simulink model "VMC_Integration"  (R2024a)
settings: Solver=FixedStepDiscrete  StartTime=0.0  StopTime=10.0  FixedStep=0.005  RelTol=1e-3
undefined symbols (not defined in the file): Degree_To_Rad_Factor
libraries: simulink x24, slpidlib x5
(part 2 of 3)

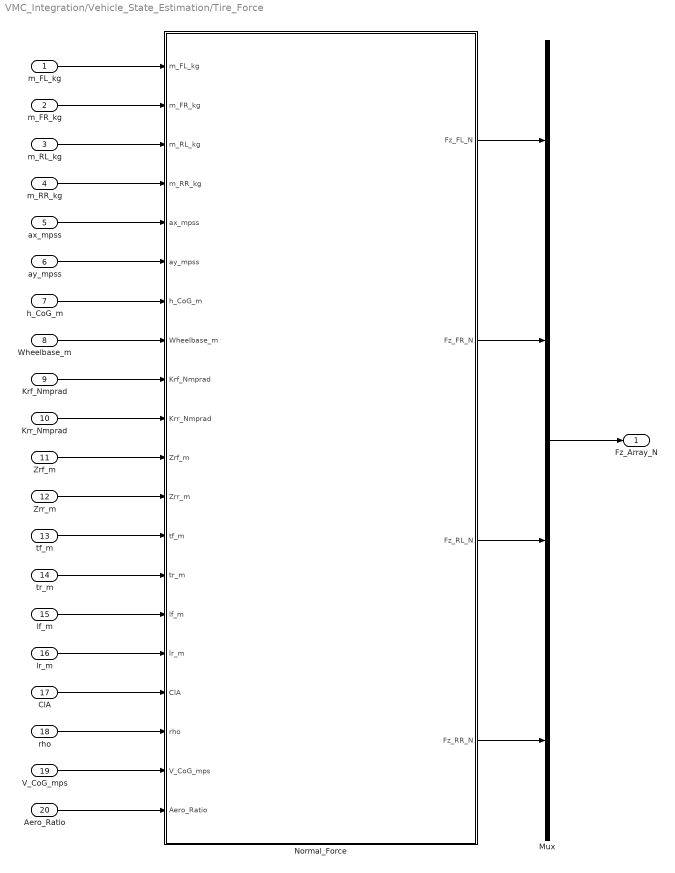
== system VMC_Integration/Vehicle_State_Estimation/Tire_Force ==
  m_FL_kg : Inport
  m_FR_kg : Inport  Port=2
  m_RL_kg : Inport  Port=3
  m_RR_kg : Inport  Port=4
  ax_mpss : Inport  Port=5
  ay_mpss : Inport  Port=6
  h_CoG_m : Inport  Port=7
  Wheelbase_m : Inport  Port=8
  Krf_Nmprad : Inport  Port=9
  Krr_Nmprad : Inport  Port=10
  Zrf_m : Inport  Port=11
  Zrr_m : Inport  Port=12
  tf_m : Inport  Port=13
  tr_m : Inport  Port=14
  lf_m : Inport  Port=15
  lr_m : Inport  Port=16
  ClA : Inport  Port=17
  rho : Inport  Port=18
  V_CoG_mps : Inport  Port=19
  Aero_Ratio : Inport  Port=20
  Mux : Mux
  Normal_Force : Subsystem
  Fz_Array_N : Outport
  wires:
  Normal_Force/1(Fz_FL_N) -> Mux/1
  Normal_Force/2(Fz_FR_N) -> Mux/2
  Normal_Force/3(Fz_RL_N) -> Mux/3
  Normal_Force/4(Fz_RR_N) -> Mux/4
  Mux/1 -> Fz_Array_N/1
  m_FL_kg/1 -> Normal_Force/1(m_FL_kg)
  m_FR_kg/1 -> Normal_Force/2(m_FR_kg)
  m_RL_kg/1 -> Normal_Force/3(m_RL_kg)
  m_RR_kg/1 -> Normal_Force/4(m_RR_kg)
  ax_mpss/1 -> Normal_Force/5(ax_mpss)
  ay_mpss/1 -> Normal_Force/6(ay_mpss)
  h_CoG_m/1 -> Normal_Force/7(h_CoG_m)
  Wheelbase_m/1 -> Normal_Force/8(Wheelbase_m)
  Krf_Nmprad/1 -> Normal_Force/9(Krf_Nmprad)
  Krr_Nmprad/1 -> Normal_Force/10(Krr_Nmprad)
  Zrf_m/1 -> Normal_Force/11(Zrf_m)
  Zrr_m/1 -> Normal_Force/12(Zrr_m)
  tf_m/1 -> Normal_Force/13(tf_m)
  tr_m/1 -> Normal_Force/14(tr_m)
  lf_m/1 -> Normal_Force/15(lf_m)
  lr_m/1 -> Normal_Force/16(lr_m)
  ClA/1 -> Normal_Force/17(ClA)
  rho/1 -> Normal_Force/18(rho)
  V_CoG_mps/1 -> Normal_Force/19(V_CoG_mps)
  Aero_Ratio/1 -> Normal_Force/20(Aero_Ratio)

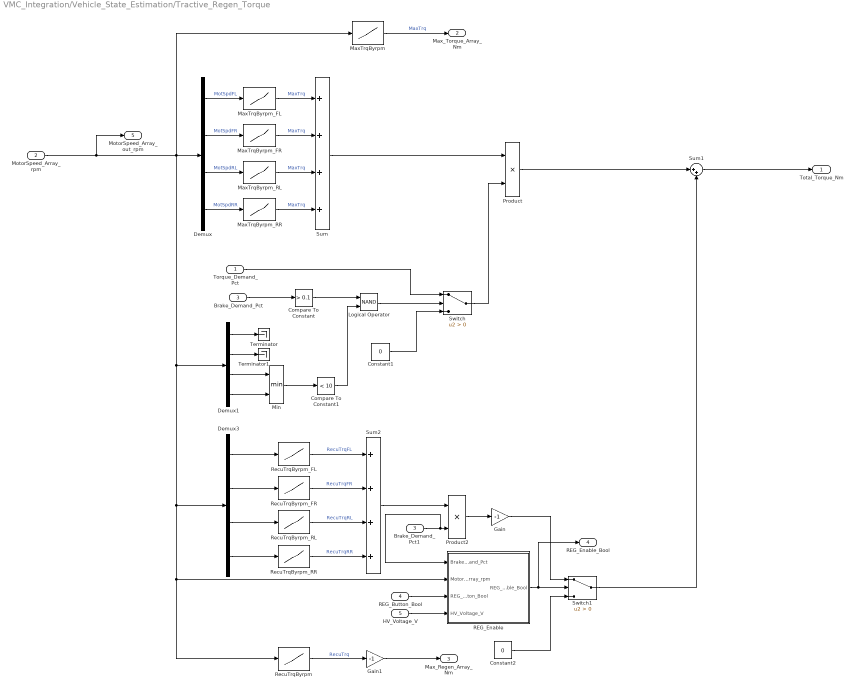
== system VMC_Integration/Vehicle_State_Estimation/Tractive_Regen_Torque ==
  Torque_Demand_Pct : Inport  OutDataTypeStr=single
  MotorSpeed_Array_rpm : Inport  Port=2  OutDataTypeStr=single
  Brake_Demand_Pct : Inport  Port=3  OutDataTypeStr=single
  REG_Button_Bool : Inport  Port=4
  HV_Voltage_V : Inport  Port=5
  Brake_Demand_Pct1 : InportShadow  Port=3  OutDataTypeStr=single
  Compare To Constant : simulink/Logic and Bit Operations/Compare To Constant  relop=>  const=0.1  OutDataTypeStr=boolean
  Compare To Constant1 : simulink/Logic and Bit Operations/Compare To Constant  relop=<  const=10  OutDataTypeStr=boolean
  Constant1 : Constant  Value=0  OutDataTypeStr=single  SampleTime=-1
  Constant2 : Constant  Value=0  OutDataTypeStr=single  SampleTime=-1
  Demux : Demux
  Demux1 : Demux
  Demux3 : Demux
  Gain : Gain  Gain=-1  ParamDataTypeStr=single  OutDataTypeStr=single
  Gain1 : Gain  Gain=-1  ParamDataTypeStr=single  OutDataTypeStr=single
  Logical Operator : Logic  Operator=NAND  AllPortsSameDT=off  OutDataTypeStr=boolean
  MaxTrqByrpm : Lookup_n-D  NumberOfTableDimensions=1  BreakpointsForDimension1=[0,16000,19999,20000]  BreakpointsForDimension1DataTypeStr=single  Table=[21,21,13,0]  TableDataTypeStr=single  IntermediateResultsDataTypeStr=single  InternalRulePriority=Speed  OutDataTypeStr=single  RndMeth=Simplest  FractionDataTypeStr=single
  MaxTrqByrpm_FL : Lookup_n-D  NumberOfTableDimensions=1  BreakpointsForDimension1=[0,16000,19999,20000]  BreakpointsForDimension1DataTypeStr=single  Table=[21,21,13,0]  TableDataTypeStr=single  IntermediateResultsDataTypeStr=single  InternalRulePriority=Speed  OutDataTypeStr=single  RndMeth=Simplest  FractionDataTypeStr=single
  MaxTrqByrpm_FR : Lookup_n-D  NumberOfTableDimensions=1  BreakpointsForDimension1=[0,16000,19999,20000]  BreakpointsForDimension1DataTypeStr=single  Table=[21,21,13,0]  TableDataTypeStr=single  IntermediateResultsDataTypeStr=single  InternalRulePriority=Speed  OutDataTypeStr=single  RndMeth=Simplest  FractionDataTypeStr=single
  MaxTrqByrpm_RL : Lookup_n-D  NumberOfTableDimensions=1  BreakpointsForDimension1=[0,16000,19999,20000]  BreakpointsForDimension1DataTypeStr=single  Table=[21,21,13,0]  TableDataTypeStr=single  IntermediateResultsDataTypeStr=single  InternalRulePriority=Speed  OutDataTypeStr=single  RndMeth=Simplest  FractionDataTypeStr=single
  MaxTrqByrpm_RR : Lookup_n-D  NumberOfTableDimensions=1  BreakpointsForDimension1=[0,16000,19999,20000]  BreakpointsForDimension1DataTypeStr=single  Table=[21,21,13,0]  TableDataTypeStr=single  IntermediateResultsDataTypeStr=single  InternalRulePriority=Speed  OutDataTypeStr=single  RndMeth=Simplest  FractionDataTypeStr=single
  Min : MinMax  Inputs=2
  Product : Product
  Product2 : Product  OutDataTypeStr=single
  REG_Enable : Subsystem
  RecuTrqByrpm : Lookup_n-D  NumberOfTableDimensions=1  BreakpointsForDimension1=[0,1500,5000,20000]  BreakpointsForDimension1DataTypeStr=single  Table=[0,0,17,17]  TableDataTypeStr=single  IntermediateResultsDataTypeStr=single  InternalRulePriority=Speed  OutDataTypeStr=single  RndMeth=Simplest  FractionDataTypeStr=single
  RecuTrqByrpm_FL : Lookup_n-D  NumberOfTableDimensions=1  BreakpointsForDimension1=[0,1500,5000,20000]  BreakpointsForDimension1DataTypeStr=single  Table=[0,0,17,17]  TableDataTypeStr=single  IntermediateResultsDataTypeStr=single  InternalRulePriority=Speed  OutDataTypeStr=single  RndMeth=Simplest  FractionDataTypeStr=single
  RecuTrqByrpm_FR : Lookup_n-D  NumberOfTableDimensions=1  BreakpointsForDimension1=[0,1500,5000,20000]  BreakpointsForDimension1DataTypeStr=single  Table=[0,0,17,17]  TableDataTypeStr=single  IntermediateResultsDataTypeStr=single  InternalRulePriority=Speed  OutDataTypeStr=single  RndMeth=Simplest  FractionDataTypeStr=single
  RecuTrqByrpm_RL : Lookup_n-D  NumberOfTableDimensions=1  BreakpointsForDimension1=[0,1500,5000,20000]  BreakpointsForDimension1DataTypeStr=single  Table=[0,0,17,17]  TableDataTypeStr=single  IntermediateResultsDataTypeStr=single  InternalRulePriority=Speed  OutDataTypeStr=single  RndMeth=Simplest  FractionDataTypeStr=single
  RecuTrqByrpm_RR : Lookup_n-D  NumberOfTableDimensions=1  BreakpointsForDimension1=[0,1500,5000,20000]  BreakpointsForDimension1DataTypeStr=single  Table=[0,0,17,17]  TableDataTypeStr=single  IntermediateResultsDataTypeStr=single  InternalRulePriority=Speed  OutDataTypeStr=single  RndMeth=Simplest  FractionDataTypeStr=single
  Sum : Sum  Inputs=++++
  Sum1 : Sum  Inputs=|++  OutDataTypeStr=single  AccumDataTypeStr=single
  Sum2 : Sum  Inputs=++++  AccumDataTypeStr=single
  Switch : Switch  Criteria=u2 > Threshold  OutDataTypeStr=single  SaturateOnIntegerOverflow=off  InputSameDT=off
  Switch1 : Switch  Criteria=u2 > Threshold  OutDataTypeStr=single  SaturateOnIntegerOverflow=off  InputSameDT=off
  Terminator : Terminator
  Terminator1 : Terminator
  Total_Torque_Nm : Outport
  Max_Torque_Array_Nm : Outport  Port=2
  Max_Regen_Array_Nm : Outport  Port=3
  REG_Enable_Bool : Outport  Port=4
  MotorSpeed_Array_out_rpm : Outport  Port=5
  wires:
  Demux/1 -> MaxTrqByrpm_FL/1  "MotSpdFL"
  Demux/2 -> MaxTrqByrpm_FR/1  "MotSpdFR"
  Demux/3 -> MaxTrqByrpm_RL/1  "MotSpdRL"
  Demux/4 -> MaxTrqByrpm_RR/1  "MotSpdRR"
  MaxTrqByrpm_FL/1 -> Sum/1  "MaxTrq"
  MaxTrqByrpm_FR/1 -> Sum/2  "MaxTrq"
  MaxTrqByrpm_RL/1 -> Sum/3  "MaxTrq"
  MaxTrqByrpm_RR/1 -> Sum/4  "MaxTrq"
  Sum/1 -> Product/1
  MaxTrqByrpm/1 -> Max_Torque_Array_Nm/1  "MaxTrq"
  Demux1/2 -> Terminator1/1
  Demux1/3 -> Min/1
  Switch/1 -> Product/2
  Constant1/1 -> Switch/3
  Logical Operator/1 -> Switch/2
  Demux1/4 -> Min/2
  Compare To Constant/1 -> Logical Operator/1
  Min/1 -> Compare To Constant1/1
  Demux1/1 -> Terminator/1
  Compare To Constant1/1 -> Logical Operator/2
  MotorSpeed_Array_rpm/1 -> MotorSpeed_Array_out_rpm/1, Demux1/1, RecuTrqByrpm/1, REG_Enable/2(MotorSpeed_Array_rpm), Demux3/1, MaxTrqByrpm/1, Demux/1
  Torque_Demand_Pct/1 -> Switch/1
  Brake_Demand_Pct/1 -> Compare To Constant/1
  REG_Enable/1(REG_Enable_Bool) -> REG_Enable_Bool/1, Switch1/2
  Gain/1 -> Switch1/1
  Brake_Demand_Pct1/1 -> REG_Enable/1(Brake_Demand_Pct), Product2/2
  Demux3/2 -> RecuTrqByrpm_FR/1
  Demux3/3 -> RecuTrqByrpm_RL/1
  Demux3/1 -> RecuTrqByrpm_FL/1
  Sum2/1 -> Product2/1
  Product2/1 -> Gain/1
  RecuTrqByrpm_RL/1 -> Sum2/3  "RecuTrqRL"
  RecuTrqByrpm_FL/1 -> Sum2/1  "RecuTrqFL"
  RecuTrqByrpm_FR/1 -> Sum2/2  "RecuTrqFR"
  Demux3/4 -> RecuTrqByrpm_RR/1
  RecuTrqByrpm_RR/1 -> Sum2/4  "RecuTrqRR"
  Constant2/1 -> Switch1/3
  REG_Button_Bool/1 -> REG_Enable/3(REG_Button_Bool)
  HV_Voltage_V/1 -> REG_Enable/4(HV_Voltage_V)
  Product/1 -> Sum1/1
  Sum1/1 -> Total_Torque_Nm/1
  Switch1/1 -> Sum1/2
  RecuTrqByrpm/1 -> Gain1/1  "RecuTrq"
  Gain1/1 -> Max_Regen_Array_Nm/1

== system VMC_Integration/Vehicle_State_Estimation/Velocity_Estimation ==
  IMU_YawRate_radps : Inport
  OS_Vx_kph : Inport  Port=2
  OS_Vy_kph : Inport  Port=3
  OS_X_Distance_m : Inport  Port=4
  OS_Y_Distance_m : Inport  Port=5
  CoG_Linear_Velocity_Calculation : MATLAB Function  TreatAsAtomicUnit=on
  CoG_Vx_mps : Outport
  CoG_Vy_mps : Outport  Port=2
  CoG_V_mps : Outport  Port=3
  OS_V_mps : Outport  Port=4
  wires:
  IMU_YawRate_radps/1 -> CoG_Linear_Velocity_Calculation/1(Actual_Yaw_Rate)
  OS_Vx_kph/1 -> CoG_Linear_Velocity_Calculation/2(OS_Vx)
  OS_Vy_kph/1 -> CoG_Linear_Velocity_Calculation/3(OS_Vy)
  OS_X_Distance_m/1 -> CoG_Linear_Velocity_Calculation/4(OS_X_Distance)
  OS_Y_Distance_m/1 -> CoG_Linear_Velocity_Calculation/5(OS_Y_Distance)
  CoG_Linear_Velocity_Calculation/1(CoG_Vx) -> CoG_Vx_mps/1
  CoG_Linear_Velocity_Calculation/2(CoG_Vy) -> CoG_Vy_mps/1
  CoG_Linear_Velocity_Calculation/3(CoG_V) -> CoG_V_mps/1
  CoG_Linear_Velocity_Calculation/4(OS_V) -> OS_V_mps/1

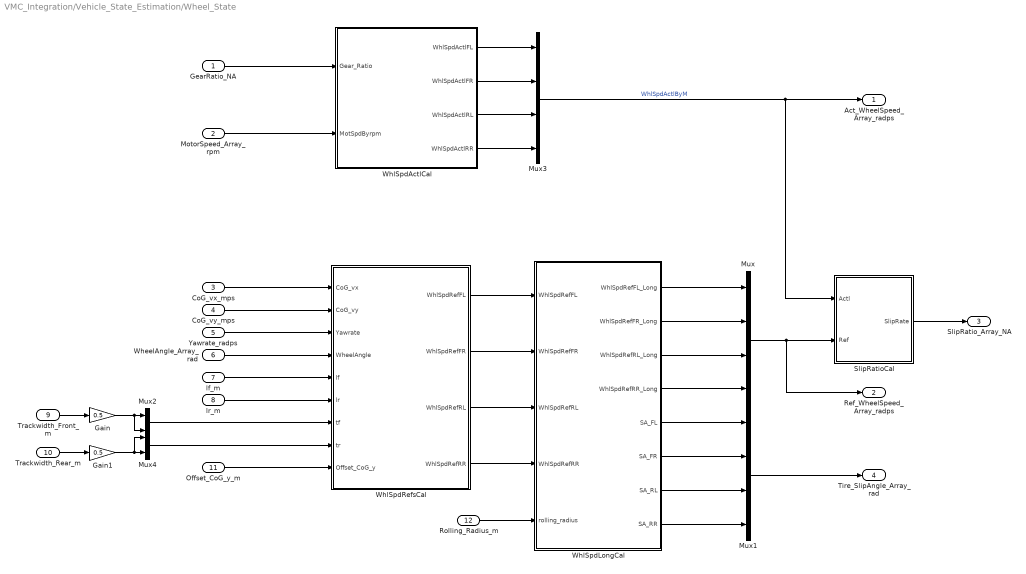
== system VMC_Integration/Vehicle_State_Estimation/Wheel_State ==
  GearRatio_NA : Inport
  MotorSpeed_Array_rpm : Inport  Port=2  PortDimensions=[4,1]
  CoG_vx_mps : Inport  Port=3
  CoG_vy_mps : Inport  Port=4
  Yawrate_radps : Inport  Port=5
  WheelAngle_Array_rad : Inport  Port=6  PortDimensions=[4,1]
  lf_m : Inport  Port=7
  lr_m : Inport  Port=8
  Trackwidth_Front_m : Inport  Port=9
  Trackwidth_Rear_m : Inport  Port=10
  Offset_CoG_y_m : Inport  Port=11
  Rolling_Radius_m : Inport  Port=12
  Gain : Gain  Gain=0.5
  Gain1 : Gain  Gain=0.5
  Mux : Mux
  Mux1 : Mux
  Mux2 : Mux  Inputs=2
  Mux3 : Mux
  Mux4 : Mux  Inputs=2
  SlipRatioCal : MATLAB Function  TreatAsAtomicUnit=on
  WhlSpdActlCal : MATLAB Function  TreatAsAtomicUnit=on
  WhlSpdLongCal : MATLAB Function  TreatAsAtomicUnit=on
  WhlSpdRefsCal : MATLAB Function  TreatAsAtomicUnit=on
  Act_WheelSpeed_Array_radps : Outport
  Ref_WheelSpeed_Array_radps : Outport  Port=2
  SlipRatio_Array_NA : Outport  Port=3
  Tire_SlipAngle_Array_rad : Outport  Port=4
  wires:
  MotorSpeed_Array_rpm/1 -> WhlSpdActlCal/2(MotSpdByrpm)
  GearRatio_NA/1 -> WhlSpdActlCal/1(Gear_Ratio)
  WhlSpdActlCal/1(WhlSpdActlFL) -> Mux3/1
  WhlSpdActlCal/2(WhlSpdActlFR) -> Mux3/2
  WhlSpdActlCal/3(WhlSpdActlRL) -> Mux3/3
  WhlSpdActlCal/4(WhlSpdActlRR) -> Mux3/4
  Mux3/1 -> SlipRatioCal/1(Actl), Act_WheelSpeed_Array_radps/1  "WhlSpdActlByM"
  WhlSpdRefsCal/1(WhlSpdRefFL) -> WhlSpdLongCal/1(WhlSpdRefFL)
  WhlSpdRefsCal/2(WhlSpdRefFR) -> WhlSpdLongCal/2(WhlSpdRefFR)
  WhlSpdRefsCal/3(WhlSpdRefRL) -> WhlSpdLongCal/3(WhlSpdRefRL)
  WhlSpdRefsCal/4(WhlSpdRefRR) -> WhlSpdLongCal/4(WhlSpdRefRR)
  WhlSpdLongCal/1(WhlSpdRefFL_Long) -> Mux/1
  WhlSpdLongCal/2(WhlSpdRefFR_Long) -> Mux/2
  WhlSpdLongCal/3(WhlSpdRefRL_Long) -> Mux/3
  WhlSpdLongCal/4(WhlSpdRefRR_Long) -> Mux/4
  WhlSpdLongCal/5(SA_FL) -> Mux1/1
  WhlSpdLongCal/6(SA_FR) -> Mux1/2
  WhlSpdLongCal/7(SA_RL) -> Mux1/3
  WhlSpdLongCal/8(SA_RR) -> Mux1/4
  Mux/1 -> Ref_WheelSpeed_Array_radps/1, SlipRatioCal/2(Ref)
  CoG_vx_mps/1 -> WhlSpdRefsCal/1(CoG_vx)
  CoG_vy_mps/1 -> WhlSpdRefsCal/2(CoG_vy)
  Yawrate_radps/1 -> WhlSpdRefsCal/3(Yawrate)
  WheelAngle_Array_rad/1 -> WhlSpdRefsCal/4(WheelAngle)
  lf_m/1 -> WhlSpdRefsCal/5(lf)
  lr_m/1 -> WhlSpdRefsCal/6(lr)
  Offset_CoG_y_m/1 -> WhlSpdRefsCal/9(Offset_CoG_y)
  Rolling_Radius_m/1 -> WhlSpdLongCal/5(rolling_radius)
  SlipRatioCal/1(SlipRate) -> SlipRatio_Array_NA/1
  Mux1/1 -> Tire_SlipAngle_Array_rad/1
  Mux2/1 -> WhlSpdRefsCal/7(tf)
  Gain/1 -> Mux2/2, Mux2/1
  Trackwidth_Front_m/1 -> Gain/1
  Gain1/1 -> Mux4/1, Mux4/2
  Mux4/1 -> WhlSpdRefsCal/8(tr)
  Trackwidth_Rear_m/1 -> Gain1/1

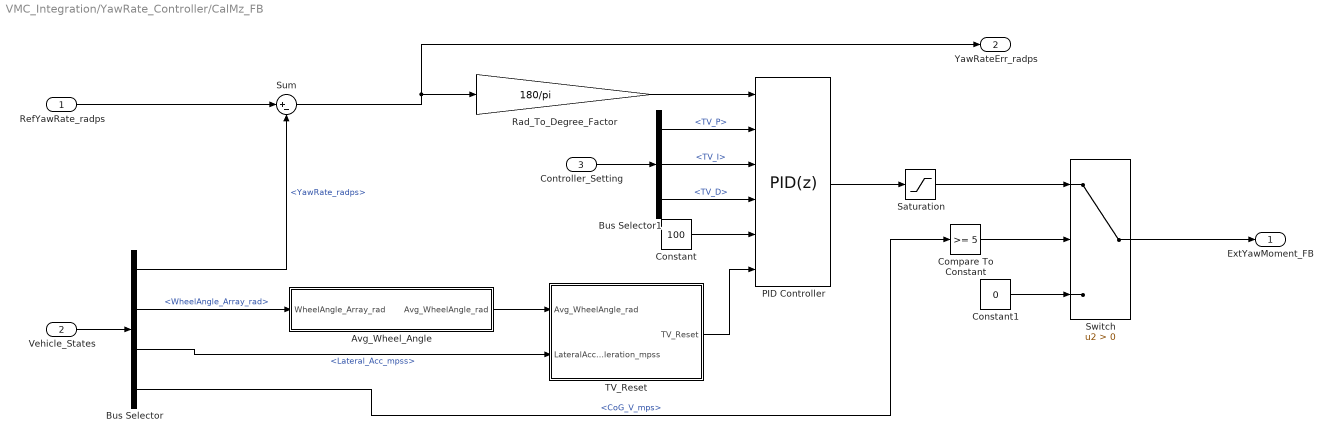
== system VMC_Integration/YawRate_Controller/CalMz_FB ==
  RefYawRate_radps : Inport
  Vehicle_States : Inport  Port=2
  Controller_Setting : Inport  Port=3
  Avg_Wheel_Angle : Subsystem
  Bus Selector : BusSelector  OutputSignals=IMU.YawRate_radps,WheelAngle.WheelAngle_Array_rad,IMU.Lateral_Acc_mpss,Vehicle_Velocity.CoG_V_mps
  Bus Selector1 : BusSelector  OutputSignals=TV_Controller.TV_PID.TV_P,TV_Controller.TV_PID.TV_I,TV_Controller.TV_PID.TV_D
  Compare To Constant : simulink/Logic and Bit Operations/Compare To Constant  relop=>=  const=5  OutDataTypeStr=boolean
  Constant : Constant  Value=100  OutDataTypeStr=single
  Constant1 : Constant  Value=0  OutDataTypeStr=single
  PID Controller : slpidlib/PID Controller  Controller=PID  Form=Parallel  TimeDomain=Discrete-time  UseExternalTs=off  SampleTime=-1  IntegratorMethod=Forward Euler  FilterMethod=Forward Euler  ControllerParametersSource=external  P=40  I=12  UseKiTs=off  D=0  UseExternalDerivativeSource=off  N=100  UseFilter=on  TunerSelectOption=Transfer Function Based (PID Tuner App)  InitialConditionSource=internal  InitialConditionForIntegrator=0  InitialConditionForFilter=0  DifferentiatorICPrevScaledInput=0  ExternalReset=rising  TrackingMode=off  Kt=1  LimitOutput=off  SatLimitsSource=internal  UpperSaturationLimit=inf  LowerSaturationLimit=-inf  LinearizeAsGain=on  AntiWindupMode=none  Kb=1  LimitIntegrator=off  UpperIntegratorSaturationLimit=inf  LowerIntegratorSaturationLimit=-inf  POutMin=[]  POutMax=[]  IOutMin=[]  IOutMax=[]  DOutMin=[]  DOutMax=[]  NOutMin=[]  NOutMax=[]  SumOutMin=[]  SumOutMax=[]  SaturationOutMin=[]  SaturationOutMax=[]  PParamMin=[]  PParamMax=[]  IParamMin=[]  IParamMax=[]  DParamMin=[]  DParamMax=[]  NParamMin=[]  NParamMax=[]  KbParamMin=[]  KbParamMax=[]  KtParamMin=[]  KtParamMax=[]  KbOutMin=[]  KbOutMax=[]  KtOutMin=[]  KtOutMax=[]  IntegratorOutMin=[]  IntegratorOutMax=[]  FilterOutMin=[]  FilterOutMax=[]  SumI1OutMin=[]  SumI1OutMax=[]  SumI2OutMin=[]  SumI2OutMax=[]  SumI3OutMin=[]  SumI3OutMax=[]  SumI4OutMin=[]  SumI4OutMax=[]  SumDOutMin=[]  SumDOutMax=[]  DifferentiatorOutMin=[]  DifferentiatorOutMax=[]  FilterDiffOutCoefMin=[]  FilterDiffOutCoefMax=[]  ReciprocalOutMin=[]  ReciprocalOutMax=[]  SumDenOutMin=[]  SumDenOutMax=[]  SumNumOutMin=[]  SumNumOutMax=[]  DivideOutMin=[]  DivideOutMax=[]  UdiffTsProdOutMin=[]  UdiffTsProdOutMax=[]  NTsProdOutMin=[]  NTsProdOutMax=[]  UintegralTsProdOutMin=[]  UintegralTsProdOutMax=[]  UngainTsProdOutMin=[]  UngainTsProdOutMax=[]  ClampingZeroOutDataTypeStr=Inherit: Inherit via back propagation  ClampingZeroOutMin=[]  ClampingZeroOutMax=[]  FilterDenConstantOutDataTypeStr=Inherit: Inherit via back propagation  FilterDenConstantOutMin=[]  FilterDenConstantOutMax=[]  PCopyOutDataTypeStr=Inherit: Inherit via back propagation  PCopyOutMin=[]  PCopyOutMax=[]  NCopyOutDataTypeStr=Inherit: Inherit via back propagation  NCopyOutMin=[]  NCopyOutMax=[]  IntegratorContinuousStateAttributes=''  IntegratorStateMustResolveToSignalObject=off  IntegratorRTWStateStorageClass=Auto  FilterContinuousStateAttributes=''  FilterStateMustResolveToSignalObject=off  FilterRTWStateStorageClass=Auto  ParallelPVariant=ExternalParameters  IdealPVariant=Disabled  IVariant=ExternalParameters  DVariant=ExternalParameters  IntegratorVariant=Discrete  SatVariant=Disabled  AWVariant=Passthrough  PCopyVariant=Disabled  TRVariant=Disabled  FdbkBlocksVariant=Forward  IdealPFdbkVariant=Disabled  SatFdbkVariant=Disabled  DerivativeFilterVariant=ForwardEulerFilter  NVariant=ExternalParameters  NCopyVariant=Disabled  FilterICVariant=InternalICsFilter  IntegratorICVariant=InternalICs  ExternalResetVariant=ExternalReset  TRSumVariant=Passthrough  SumFdbkVariant=Disabled  SumVariant=Sum_PID  TsampFilterVariant=InternalTs  TsampNgainVariant=Passthrough  TsampIntegralVariant=Disabled_SignalSpec  ExternalSaturationOutDataTypeStr=Inherit: Same as second input  DerivativeSourceVariant=ErrorSignal
  Rad_To_Degree_Factor : Gain  Gain=180/pi  ParamDataTypeStr=single
  Saturation : Saturate  UpperLimit=1500  LowerLimit=-1500  OutDataTypeStr=single
  Sum : Sum  Inputs=|+-  OutDataTypeStr=single  AccumDataTypeStr=single
  Switch : Switch  Criteria=u2 > Threshold  SaturateOnIntegerOverflow=off  InputSameDT=off
  TV_Reset : Subsystem
  ExtYawMoment_FB : Outport
  YawRateErr_radps : Outport  Port=2
  wires:
  PID Controller/1 -> Saturation/1
  Sum/1 -> Rad_To_Degree_Factor/1, YawRateErr_radps/1
  Rad_To_Degree_Factor/1 -> PID Controller/1
  TV_Reset/1(TV_Reset) -> PID Controller/6
  Bus Selector1/2 -> PID Controller/3  "<TV_I>"
  Bus Selector1/3 -> PID Controller/4  "<TV_D>"
  Bus Selector1/1 -> PID Controller/2  "<TV_P>"
  Constant/1 -> PID Controller/5
  Controller_Setting/1 -> Bus Selector1/1
  RefYawRate_radps/1 -> Sum/1
  Vehicle_States/1 -> Bus Selector/1
  Bus Selector/1 -> Sum/2  "<YawRate_radps>"
  Bus Selector/3 -> TV_Reset/2(LateralAcceleration_mpss)  "<Lateral_Acc_mpss>"
  Avg_Wheel_Angle/1(Avg_WheelAngle_rad) -> TV_Reset/1(Avg_WheelAngle_rad)
  Bus Selector/2 -> Avg_Wheel_Angle/1(WheelAngle_Array_rad)  "<WheelAngle_Array_rad>"
  Saturation/1 -> Switch/1
  Switch/1 -> ExtYawMoment_FB/1
  Constant1/1 -> Switch/3
  Compare To Constant/1 -> Switch/2
  Bus Selector/4 -> Compare To Constant/1  "<CoG_V_mps>"

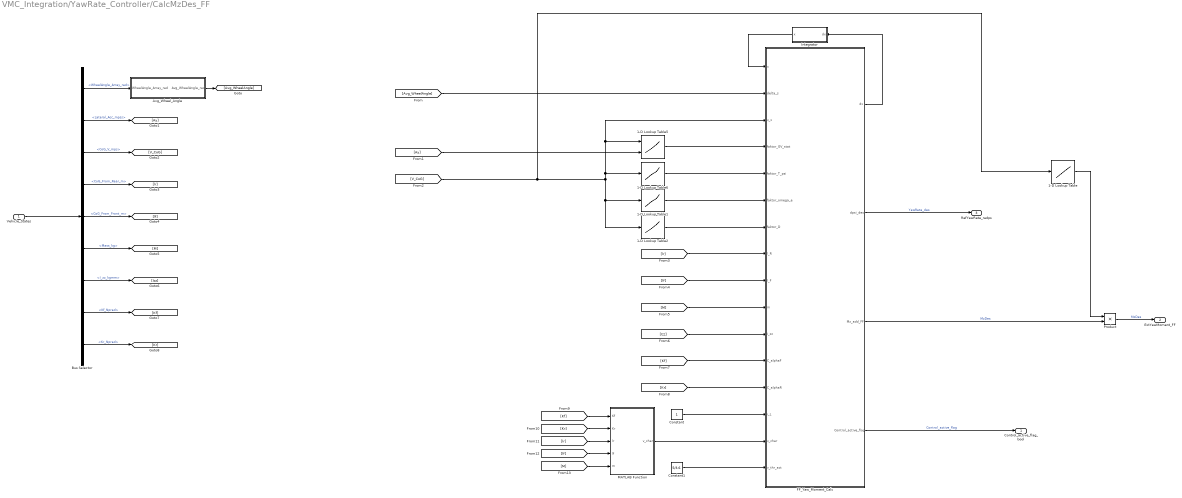
== system VMC_Integration/YawRate_Controller/CalcMzDes_FF ==
  Vehicle_States : Inport
  1-D Lookup Table : Lookup_n-D  NumberOfTableDimensions=1  BreakpointsForDimension1=[0, 5/3.6, 10/3.6, 100]  BreakpointsForDimension1DataTypeStr=single  Table=[0 0 1 1]  TableDataTypeStr=single  IntermediateResultsDataTypeStr=single  InternalRulePriority=Speed  OutDataTypeStr=single  RndMeth=Simplest  FractionDataTypeStr=single
  1-D Lookup Table1 : Lookup_n-D  NumberOfTableDimensions=1  BreakpointsForDimension1=[0, 200]  BreakpointsForDimension1DataTypeStr=single  Table=[1,1]  TableDataTypeStr=single  IntermediateResultsDataTypeStr=single  InternalRulePriority=Speed  OutDataTypeStr=single  RndMeth=Simplest  FractionDataTypeStr=single
  1-D Lookup Table2 : Lookup_n-D  NumberOfTableDimensions=1  BreakpointsForDimension1=[0, 200]  BreakpointsForDimension1DataTypeStr=single  Table=[1,1]  TableDataTypeStr=single  IntermediateResultsDataTypeStr=single  InternalRulePriority=Speed  OutDataTypeStr=single  RndMeth=Simplest  FractionDataTypeStr=single
  1-D Lookup Table5 : Lookup_n-D  BreakpointsForDimension1=[0, 200]  BreakpointsForDimension2=[-20, 20]  BreakpointsForDimension1DataTypeStr=single  BreakpointsForDimension2DataTypeStr=single  Table=[1.1,1.1;1.1,1.1]  TableDataTypeStr=single  IntermediateResultsDataTypeStr=single  InternalRulePriority=Speed  OutDataTypeStr=single  RndMeth=Simplest  FractionDataTypeStr=single
      settings: InputPortMap=u0,u1
  1-D Lookup Table6 : Lookup_n-D  NumberOfTableDimensions=1  BreakpointsForDimension1=[0, 200]  BreakpointsForDimension1DataTypeStr=single  Table=[1,1]  TableDataTypeStr=single  IntermediateResultsDataTypeStr=single  InternalRulePriority=Speed  OutDataTypeStr=single  RndMeth=Simplest  FractionDataTypeStr=single
  Avg_Wheel_Angle : Subsystem
  Bus Selector : BusSelector  OutputSignals=WheelAngle.WheelAngle_Array_rad,IMU.Lateral_Acc_mpss,Vehicle_Velocity.CoG_V_mps,Vehicle_Static_Parameter.CoG_From_Rear_m,Vehicle_Static_Parameter.CoG_From_Front_m,Vehicle_Static_Parameter.Mass_kg,Vehicle_Static_Parameter.I_zz_kgmm,Vehicle_Static_Parameter.Kf_Nprad,Vehicle_Static_Parameter.Kr_Nprad
  Constant : Constant  OutDataTypeStr=single
  Constant1 : Constant  Value=5/3.6  OutDataTypeStr=single
  FF_Yaw_Moment_Calc : MATLAB Function  TreatAsAtomicUnit=on
  Integrator : Subsystem
  MATLAB Function : MATLAB Function  TreatAsAtomicUnit=on
  Product : Product
  Control_active_flag_bool : Outport
  ExtYawMoment_FF : Outport  Port=2
  RefYawRate_radps : Outport  Port=3
  wires:
  Integrator/1(x) -> FF_Yaw_Moment_Calc/1(x)
  [Ay] -> 1-D Lookup Table5/2
  FF_Yaw_Moment_Calc/1(dx) -> Integrator/1(dx)
  FF_Yaw_Moment_Calc/3(Mz_add_FF) -> Product/2  "MzDes"
  FF_Yaw_Moment_Calc/2(dpsi_des) -> RefYawRate_radps/1  "YawRate_des"
  [lr] -> FF_Yaw_Moment_Calc/8(l_R)
  [lf] -> FF_Yaw_Moment_Calc/9(l_F)
  [M] -> FF_Yaw_Moment_Calc/10(m)
  [Izz] -> FF_Yaw_Moment_Calc/11(I_zz)
  [Kf] -> FF_Yaw_Moment_Calc/12(C_alphaF)
  [Kr] -> FF_Yaw_Moment_Calc/13(C_alphaR)
  FF_Yaw_Moment_Calc/4(Control_active_flag) -> Control_active_flag_bool/1  "Control_active_flag"
  [V_CoG] -> 1-D Lookup Table/1, FF_Yaw_Moment_Calc/3(v_x), 1-D Lookup Table5/1, 1-D Lookup Table6/1, 1-D Lookup Table2/1, 1-D Lookup Table1/1
  [Avg_WheelAngle] -> FF_Yaw_Moment_Calc/2(delta_s)
  1-D Lookup Table5/1 -> FF_Yaw_Moment_Calc/4(faktor_GV_stat)
  1-D Lookup Table6/1 -> FF_Yaw_Moment_Calc/5(faktor_T_psi)
  1-D Lookup Table1/1 -> FF_Yaw_Moment_Calc/6(faktor_omega_e)
  1-D Lookup Table2/1 -> FF_Yaw_Moment_Calc/7(faktor_D)
  1-D Lookup Table/1 -> Product/1
  Product/1 -> ExtYawMoment_FF/1  "MzDes"
  Vehicle_States/1 -> Bus Selector/1
  Bus Selector/1 -> Avg_Wheel_Angle/1(WheelAngle_Array_rad)  "<WheelAngle_Array_rad>"
  Avg_Wheel_Angle/1(Avg_WheelAngle_rad) -> [Avg_WheelAngle]
  Bus Selector/2 -> [Ay]  "<Lateral_Acc_mpss>"
  Bus Selector/3 -> [V_CoG]  "<CoG_V_mps>"
  Bus Selector/4 -> [lr]  "<CoG_From_Rear_m>"
  Bus Selector/5 -> [lf]  "<CoG_From_Front_m>"
  Bus Selector/6 -> [M]  "<Mass_kg>"
  Bus Selector/7 -> [Izz]  "<I_zz_kgmm>"
  Bus Selector/8 -> [Kf]  "<Kf_Nprad>"
  Bus Selector/9 -> [Kr]  "<Kr_Nprad>"
  Constant/1 -> FF_Yaw_Moment_Calc/14(i_L)
  MATLAB Function/1(v_char) -> FF_Yaw_Moment_Calc/15(v_char)
  Constant1/1 -> FF_Yaw_Moment_Calc/16(v_thr_act)
  [Kf] -> MATLAB Function/1(Kf)
  [Kr] -> MATLAB Function/2(Kr)
  [lr] -> MATLAB Function/3(lr)
  [lf] -> MATLAB Function/4(lf)
  [M] -> MATLAB Function/5(m)

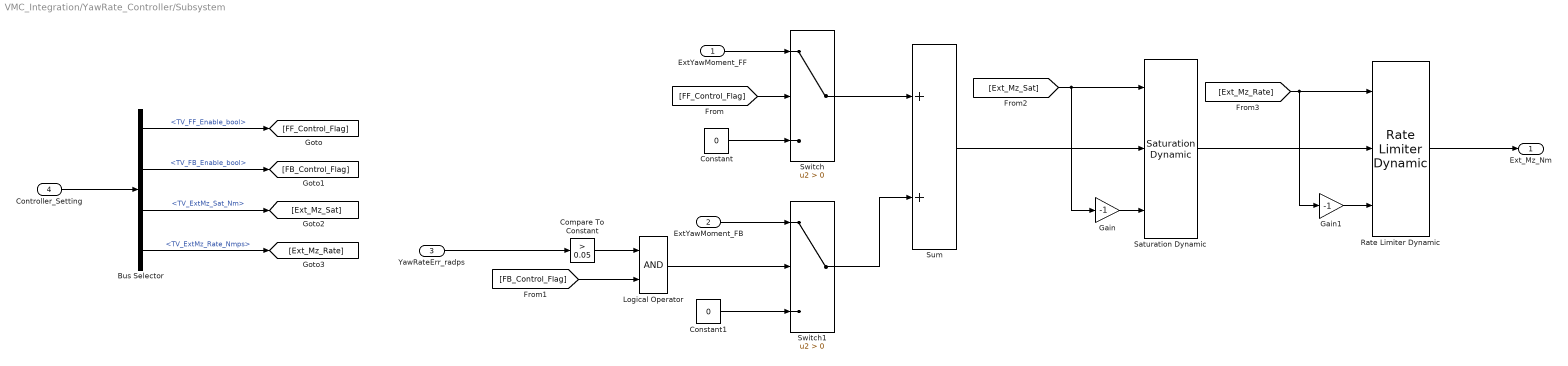
== system VMC_Integration/YawRate_Controller/Subsystem ==
  ExtYawMoment_FF : Inport
  ExtYawMoment_FB : Inport  Port=2
  YawRateErr_radps : Inport  Port=3
  Controller_Setting : Inport  Port=4
  Bus Selector : BusSelector  OutputSignals=TV_Controller.TV_FF_Enable_bool,TV_Controller.TV_FB_Enable_bool,TV_Controller.TV_ExtMz_Sat_Nm,TV_Controller.TV_ExtMz_Rate_Nmps
  Compare To Constant : simulink/Logic and Bit Operations/Compare To Constant  relop=>  const=0.05  OutDataTypeStr=boolean
  Constant : Constant  Value=0  OutDataTypeStr=single
  Constant1 : Constant  Value=0  OutDataTypeStr=single
  Gain : Gain  Gain=-1
  Gain1 : Gain  Gain=-1
  Logical Operator : Logic  AllPortsSameDT=off  OutDataTypeStr=boolean
  Rate Limiter Dynamic : simulink/Discontinuities/Rate Limiter Dynamic
  Saturation Dynamic : simulink/Discontinuities/Saturation Dynamic  OutMin=[]  OutMax=[]  OutDataTypeStr=Inherit: Same as second input  OutDataType=fixdt(1, 16)  OutScaling=2^-10  DoSatur=off
  Sum : Sum
  Switch : Switch  Criteria=u2 > Threshold  SaturateOnIntegerOverflow=off  InputSameDT=off
  Switch1 : Switch  Criteria=u2 > Threshold  SaturateOnIntegerOverflow=off  InputSameDT=off
  Ext_Mz_Nm : Outport
  wires:
  ExtYawMoment_FF/1 -> Switch/1
  [FF_Control_Flag] -> Switch/2
  Constant/1 -> Switch/3
  ExtYawMoment_FB/1 -> Switch1/1
  YawRateErr_radps/1 -> Compare To Constant/1
  Logical Operator/1 -> Switch1/2
  Compare To Constant/1 -> Logical Operator/1
  [FB_Control_Flag] -> Logical Operator/2
  Constant1/1 -> Switch1/3
  Switch/1 -> Sum/1
  Switch1/1 -> Sum/2
  Sum/1 -> Saturation Dynamic/2
  Rate Limiter Dynamic/1 -> Ext_Mz_Nm/1
  Saturation Dynamic/1 -> Rate Limiter Dynamic/2
  [Ext_Mz_Sat] -> Gain/1, Saturation Dynamic/1
  Gain/1 -> Saturation Dynamic/3
  [Ext_Mz_Rate] -> Gain1/1, Rate Limiter Dynamic/1
  Gain1/1 -> Rate Limiter Dynamic/3
  Controller_Setting/1 -> Bus Selector/1
  Bus Selector/1 -> [FF_Control_Flag]  "<TV_FF_Enable_bool>"
  Bus Selector/2 -> [FB_Control_Flag]  "<TV_FB_Enable_bool>"
  Bus Selector/3 -> [Ext_Mz_Sat]  "<TV_ExtMz_Sat_Nm>"
  Bus Selector/4 -> [Ext_Mz_Rate]  "<TV_ExtMz_Rate_Nmps>"

== system VMC_Integration/Traction_Control/LSD_Enable/LSD_EnableFL ==
  BrkDmd : Inport
  WhlSpdActlFL : Inport  Port=2
  WhlSpdRefFL : Inport  Port=3
  Compare To Constant1 : simulink/Logic and Bit Operations/Compare To Constant  relop=<  const=0.1  OutDataTypeStr=boolean
  Compare To Constant3 : simulink/Logic and Bit Operations/Compare To Constant  relop=>=  const=10  OutDataTypeStr=boolean
  Logical Operator : Logic  Inputs=3  AllPortsSameDT=off  OutDataTypeStr=boolean
  SlipJudge : simulink/Logic and Bit Operations/Compare To Constant  relop=>=  const=0.1  OutDataTypeStr=boolean
  LSD_EnableFL : Outport  VectorParamsAs1DForOutWhenUnconnected=off
  wires:
  WhlSpdActlFL/1 -> Compare To Constant3/1
  WhlSpdRefFL/1 -> SlipJudge/1  "SlipRateFL"
  Compare To Constant1/1 -> Logical Operator/1
  BrkDmd/1 -> Compare To Constant1/1
  Logical Operator/1 -> LSD_EnableFL/1  "LSD_EnableFL"
  Compare To Constant3/1 -> Logical Operator/2
  SlipJudge/1 -> Logical Operator/3

== system VMC_Integration/Traction_Control/LSD_Enable/LSD_EnableFR ==
  BrkDmd : Inport
  WhlSpdActlFR : Inport  Port=2
  WhlSpdRefFR : Inport  Port=3
  Compare To Constant1 : simulink/Logic and Bit Operations/Compare To Constant  relop=<  const=0.1  OutDataTypeStr=boolean
  Compare To Constant3 : simulink/Logic and Bit Operations/Compare To Constant  relop=>=  const=10  OutDataTypeStr=boolean
  Logical Operator : Logic  Inputs=3  AllPortsSameDT=off  OutDataTypeStr=boolean
  SlipJudge : simulink/Logic and Bit Operations/Compare To Constant  relop=>=  const=0.1  OutDataTypeStr=boolean
  LSD_EnableFL : Outport  VectorParamsAs1DForOutWhenUnconnected=off
  wires:
  SlipJudge/1 -> Logical Operator/3
  Compare To Constant3/1 -> Logical Operator/2
  Logical Operator/1 -> LSD_EnableFL/1  "LSD_EnableFL"
  BrkDmd/1 -> Compare To Constant1/1
  Compare To Constant1/1 -> Logical Operator/1
  WhlSpdRefFR/1 -> SlipJudge/1  "SlipRateFR"
  WhlSpdActlFR/1 -> Compare To Constant3/1

== system VMC_Integration/Traction_Control/LSD_Enable/LSD_EnableRL ==
  BrkDmd : Inport
  WhlSpdActlRL : Inport  Port=2
  WhlSpdRefRL : Inport  Port=3
  Compare To Constant1 : simulink/Logic and Bit Operations/Compare To Constant  relop=<  const=0.1  OutDataTypeStr=boolean
  Compare To Constant3 : simulink/Logic and Bit Operations/Compare To Constant  relop=>=  const=10  OutDataTypeStr=boolean
  Logical Operator : Logic  Inputs=3  AllPortsSameDT=off  OutDataTypeStr=boolean
  SlipJudge : simulink/Logic and Bit Operations/Compare To Constant  relop=>=  const=0.1  OutDataTypeStr=boolean
  LSD_EnableFL : Outport  VectorParamsAs1DForOutWhenUnconnected=off
  wires:
  WhlSpdActlRL/1 -> Compare To Constant3/1
  WhlSpdRefRL/1 -> SlipJudge/1  "SlipRateRL"
  Compare To Constant1/1 -> Logical Operator/1
  BrkDmd/1 -> Compare To Constant1/1
  Logical Operator/1 -> LSD_EnableFL/1  "LSD_EnableFL"
  Compare To Constant3/1 -> Logical Operator/2
  SlipJudge/1 -> Logical Operator/3

== system VMC_Integration/Traction_Control/LSD_Enable/LSD_EnableRR  ==
  BrkDmd : Inport
  WhlSpdActlRR : Inport  Port=2
  WhlSpdRefRR : Inport  Port=3
  Compare To Constant1 : simulink/Logic and Bit Operations/Compare To Constant  relop=<  const=0.1  OutDataTypeStr=boolean
  Compare To Constant3 : simulink/Logic and Bit Operations/Compare To Constant  relop=>=  const=10  OutDataTypeStr=boolean
  Logical Operator : Logic  Inputs=3  AllPortsSameDT=off  OutDataTypeStr=boolean
  SlipJudge : simulink/Logic and Bit Operations/Compare To Constant  relop=>=  const=0.1  OutDataTypeStr=boolean
  LSD_EnableFL : Outport  VectorParamsAs1DForOutWhenUnconnected=off
  wires:
  SlipJudge/1 -> Logical Operator/3
  Compare To Constant3/1 -> Logical Operator/2
  Logical Operator/1 -> LSD_EnableFL/1  "LSD_EnableFL"
  BrkDmd/1 -> Compare To Constant1/1
  Compare To Constant1/1 -> Logical Operator/1
  WhlSpdRefRR/1 -> SlipJudge/1  "SlipRateRR"
  WhlSpdActlRR/1 -> Compare To Constant3/1

== system VMC_Integration/Traction_Control/LimitedSlipDifferential/LSD_Ctrl ==
  Vehicle_States : Inport
  LSD_Enable : Inport  Port=2
  Bus Creator{,1..3} (4 alike) : BusCreator  Inputs=3
  Bus Selector : BusSelector  OutputSignals=Wheel.Ref_WheelSpeed_Array_radps,Vehicle_Static_Parameter.Gear_Ratio_NA,Torque_Demand.MotorSpeed_Array_rpm
  Constant : Constant  Value=30 / pi  OutDataTypeStr=single
  Demux : Demux
  Demux1 : Demux
  Demux2 : Demux
  Divide : Product  Inputs=***  OutDataTypeStr=single
  LSD_CtrlFL : Outport
  LSD_CtrlFR : Outport  Port=2
  LSD_CtrlRL : Outport  Port=3
  LSD_CtrlRR : Outport  Port=4
  wires:
  Constant/1 -> Divide/3
  Demux2/4 -> Bus Creator3/1  "MotSpdRefByrpmRR"
  Divide/1 -> Demux2/1  "MotSpdRefbyrpm"
  Demux2/1 -> Bus Creator/1  "MotSpdRefByrpmFL"
  Demux2/2 -> Bus Creator1/1  "MotSpdRefByrpmFR"
  Demux2/3 -> Bus Creator2/1  "MotSpdRefByrpmRL"
  Demux1/4 -> Bus Creator3/2  "MotSpdActlByrpmRR"
  Demux1/2 -> Bus Creator1/2  "MotSpdActlByrpmFR"
  Demux1/3 -> Bus Creator2/2  "MotSpdActlByrpmRL"
  Demux1/1 -> Bus Creator/2  "MotSpdActlByrpmFL"
  Demux/1 -> Bus Creator/3  "LSD_EnableFL"
  Demux/2 -> Bus Creator1/3  "LSD_EnableFR"
  Demux/3 -> Bus Creator2/3  "LSD_EnableRL"
  Demux/4 -> Bus Creator3/3  "LSD_EnableRR"
  Bus Creator/1 -> LSD_CtrlFL/1  "LSD_CtrlFL"
  Bus Creator1/1 -> LSD_CtrlFR/1  "LSD_CtrlFR"
  Bus Creator2/1 -> LSD_CtrlRL/1  "LSD_CtrlRL"
  Bus Creator3/1 -> LSD_CtrlRR/1  "LSD_CtrlRR"
  Bus Selector/1 -> Divide/1  "<Ref_WheelSpeed_Array_radps>"
  LSD_Enable/1 -> Demux/1
  Bus Selector/3 -> Demux1/1  "<MotorSpeed_Array_rpm>"
  Vehicle_States/1 -> Bus Selector/1
  Bus Selector/2 -> Divide/2  "<Gear_Ratio_NA>"

== system VMC_Integration/Traction_Control/LimitedSlipDifferential/PID_CtrlFL ==
  LSD_CtrlFL : Inport
  EDS_TrqFL : Inport  Port=2
  PID_Setting : Inport  Port=3
  Add1 : Sum  AccumDataTypeStr=single
  Bus Selector : BusSelector  OutputSignals=MotSpdRefByrpmFL,MotSpdActlByrpmFL,LSD_EnableFL
  Demux : Demux  Outputs=5
  Gain : Gain  Gain=0.001  ParamDataTypeStr=single  OutDataTypeStr=single
  PID Controller : slpidlib/PID Controller  Controller=PID  Form=Parallel  TimeDomain=Discrete-time  UseExternalTs=off  SampleTime=-1  IntegratorMethod=Forward Euler  FilterMethod=Forward Euler  ControllerParametersSource=external  P=500  I=0  UseKiTs=off  D=0  UseExternalDerivativeSource=off  N=100  UseFilter=on  TunerSelectOption=Transfer Function Based (PID Tuner App)  InitialConditionSource=internal  InitialConditionForIntegrator=0  InitialConditionForFilter=0  DifferentiatorICPrevScaledInput=0  ExternalReset=rising  TrackingMode=off  Kt=1  LimitOutput=off  SatLimitsSource=internal  UpperSaturationLimit=inf  LowerSaturationLimit=-inf  LinearizeAsGain=on  AntiWindupMode=none  Kb=1  LimitIntegrator=off  UpperIntegratorSaturationLimit=inf  LowerIntegratorSaturationLimit=-inf  PGainOutDataTypeStr=single  PProdOutDataTypeStr=single  POutMin=[]  POutMax=[]  IGainOutDataTypeStr=single  IProdOutDataTypeStr=single  IOutMin=[]  IOutMax=[]  DGainOutDataTypeStr=single  DProdOutDataTypeStr=single  DOutMin=[]  DOutMax=[]  NGainOutDataTypeStr=single  NProdOutDataTypeStr=single  NOutMin=[]  NOutMax=[]  SumOutDataTypeStr=single  SumOutMin=[]  SumOutMax=[]  SaturationOutMin=[]  SaturationOutMax=[]  PParamMin=[]  PParamMax=[]  IParamMin=[]  IParamMax=[]  DParamMin=[]  DParamMax=[]  NParamMin=[]  NParamMax=[]  KbParamMin=[]  KbParamMax=[]  KtParamMin=[]  KtParamMax=[]  KbOutMin=[]  KbOutMax=[]  KtOutMin=[]  KtOutMax=[]  IntegratorOutMin=[]  IntegratorOutMax=[]  FilterOutMin=[]  FilterOutMax=[]  SumI1OutMin=[]  SumI1OutMax=[]  SumI2OutMin=[]  SumI2OutMax=[]  SumI3OutMin=[]  SumI3OutMax=[]  SumI4OutMin=[]  SumI4OutMax=[]  SumDOutMin=[]  SumDOutMax=[]  DifferentiatorOutMin=[]  DifferentiatorOutMax=[]  FilterDiffOutCoefMin=[]  FilterDiffOutCoefMax=[]  ReciprocalOutMin=[]  ReciprocalOutMax=[]  SumDenOutMin=[]  SumDenOutMax=[]  SumNumOutMin=[]  SumNumOutMax=[]  DivideOutMin=[]  DivideOutMax=[]  UdiffTsProdOutMin=[]  UdiffTsProdOutMax=[]  NTsProdOutMin=[]  NTsProdOutMax=[]  UintegralTsProdOutMin=[]  UintegralTsProdOutMax=[]  UngainTsProdOutMin=[]  UngainTsProdOutMax=[]  ClampingZeroOutDataTypeStr=Inherit: Inherit via back propagation  ClampingZeroOutMin=[]  ClampingZeroOutMax=[]  FilterDenConstantOutDataTypeStr=Inherit: Inherit via back propagation  FilterDenConstantOutMin=[]  FilterDenConstantOutMax=[]  PCopyOutDataTypeStr=Inherit: Inherit via back propagation  PCopyOutMin=[]  PCopyOutMax=[]  NCopyOutDataTypeStr=Inherit: Inherit via back propagation  NCopyOutMin=[]  NCopyOutMax=[]  IntegratorContinuousStateAttributes=''  IntegratorStateMustResolveToSignalObject=off  IntegratorRTWStateStorageClass=Auto  FilterContinuousStateAttributes=''  FilterStateMustResolveToSignalObject=off  FilterRTWStateStorageClass=Auto  ParallelPVariant=ExternalParameters  IdealPVariant=Disabled  IVariant=ExternalParameters  DVariant=ExternalParameters  IntegratorVariant=Discrete  SatVariant=Disabled  AWVariant=Passthrough  PCopyVariant=Disabled  TRVariant=Disabled  FdbkBlocksVariant=Forward  IdealPFdbkVariant=Disabled  SatFdbkVariant=Disabled  DerivativeFilterVariant=ForwardEulerFilter  NVariant=ExternalParameters  NCopyVariant=Disabled  FilterICVariant=InternalICsFilter  IntegratorICVariant=InternalICs  ExternalResetVariant=ExternalReset  TRSumVariant=Passthrough  SumFdbkVariant=Disabled  SumVariant=Sum_PID  TsampFilterVariant=InternalTs  TsampNgainVariant=Passthrough  TsampIntegralVariant=Disabled_SignalSpec  ExternalSaturationOutDataTypeStr=Inherit: Same as second input  DerivativeSourceVariant=ErrorSignal
  Saturation1 : Saturate  UpperLimit=0  LowerLimit=-10
  SpdDiffFL : Sum  Inputs=+-  OutDataTypeStr=single  AccumDataTypeStr=single
  Switch : Switch  Criteria=u2 > Threshold  OutDataTypeStr=single  SaturateOnIntegerOverflow=off  InputSameDT=off
  LSD_TrqFL : Outport  VectorParamsAs1DForOutWhenUnconnected=off
  wires:
  Add1/1 -> Switch/1  "LSDTrqFL"
  EDS_TrqFL/1 -> Add1/2, Switch/3
  LSD_CtrlFL/1 -> Bus Selector/1
  Bus Selector/1 -> SpdDiffFL/1  "<MotSpdRefByrpmFL>"
  Bus Selector/2 -> SpdDiffFL/2  "<MotSpdActlByrpmFL>"
  Bus Selector/3 -> Switch/2  "<LSD_EnableFL>"
  Switch/1 -> LSD_TrqFL/1  "LSD_TrqFL"
  Demux/4 -> PID Controller/5  "N"
  Demux/1 -> PID Controller/2  "P"
  PID Controller/1 -> Saturation1/1  "TrqModFL"
  Demux/2 -> PID Controller/3  "I"
  Demux/3 -> PID Controller/4  "D"
  Demux/5 -> PID Controller/6  "PID_Reset"
  PID_Setting/1 -> Demux/1
  Gain/1 -> PID Controller/1  "SpdDiffFLScaled"
  SpdDiffFL/1 -> Gain/1  "SpdDiffFL"
  Saturation1/1 -> Add1/1

== system VMC_Integration/Traction_Control/LimitedSlipDifferential/PID_CtrlFR ==
  LSD_CtrlFR : Inport
  EDS_TrqFR : Inport  Port=2
  PID_Setting : Inport  Port=3
  Add1 : Sum  AccumDataTypeStr=single
  Bus Selector : BusSelector  OutputSignals=MotSpdRefByrpmFR,MotSpdActlByrpmFR,LSD_EnableFR
  Demux : Demux  Outputs=5
  Gain : Gain  Gain=0.001  ParamDataTypeStr=single  OutDataTypeStr=single
  PID Controller : slpidlib/PID Controller  Controller=PID  Form=Parallel  TimeDomain=Discrete-time  UseExternalTs=off  SampleTime=-1  IntegratorMethod=Forward Euler  FilterMethod=Forward Euler  ControllerParametersSource=external  P=500  I=0  UseKiTs=off  D=0  UseExternalDerivativeSource=off  N=100  UseFilter=on  TunerSelectOption=Transfer Function Based (PID Tuner App)  InitialConditionSource=internal  InitialConditionForIntegrator=0  InitialConditionForFilter=0  DifferentiatorICPrevScaledInput=0  ExternalReset=rising  TrackingMode=off  Kt=1  LimitOutput=off  SatLimitsSource=internal  UpperSaturationLimit=inf  LowerSaturationLimit=-inf  LinearizeAsGain=on  AntiWindupMode=none  Kb=1  LimitIntegrator=off  UpperIntegratorSaturationLimit=inf  LowerIntegratorSaturationLimit=-inf  PGainOutDataTypeStr=single  PProdOutDataTypeStr=single  POutMin=[]  POutMax=[]  IGainOutDataTypeStr=single  IProdOutDataTypeStr=single  IOutMin=[]  IOutMax=[]  DGainOutDataTypeStr=single  DProdOutDataTypeStr=single  DOutMin=[]  DOutMax=[]  NGainOutDataTypeStr=single  NProdOutDataTypeStr=single  NOutMin=[]  NOutMax=[]  SumOutDataTypeStr=single  SumOutMin=[]  SumOutMax=[]  SaturationOutMin=[]  SaturationOutMax=[]  PParamMin=[]  PParamMax=[]  IParamMin=[]  IParamMax=[]  DParamMin=[]  DParamMax=[]  NParamMin=[]  NParamMax=[]  KbParamMin=[]  KbParamMax=[]  KtParamMin=[]  KtParamMax=[]  KbOutMin=[]  KbOutMax=[]  KtOutMin=[]  KtOutMax=[]  IntegratorOutMin=[]  IntegratorOutMax=[]  FilterOutMin=[]  FilterOutMax=[]  SumI1OutMin=[]  SumI1OutMax=[]  SumI2OutMin=[]  SumI2OutMax=[]  SumI3OutMin=[]  SumI3OutMax=[]  SumI4OutMin=[]  SumI4OutMax=[]  SumDOutMin=[]  SumDOutMax=[]  DifferentiatorOutMin=[]  DifferentiatorOutMax=[]  FilterDiffOutCoefMin=[]  FilterDiffOutCoefMax=[]  ReciprocalOutMin=[]  ReciprocalOutMax=[]  SumDenOutMin=[]  SumDenOutMax=[]  SumNumOutMin=[]  SumNumOutMax=[]  DivideOutMin=[]  DivideOutMax=[]  UdiffTsProdOutMin=[]  UdiffTsProdOutMax=[]  NTsProdOutMin=[]  NTsProdOutMax=[]  UintegralTsProdOutMin=[]  UintegralTsProdOutMax=[]  UngainTsProdOutMin=[]  UngainTsProdOutMax=[]  ClampingZeroOutDataTypeStr=Inherit: Inherit via back propagation  ClampingZeroOutMin=[]  ClampingZeroOutMax=[]  FilterDenConstantOutDataTypeStr=Inherit: Inherit via back propagation  FilterDenConstantOutMin=[]  FilterDenConstantOutMax=[]  PCopyOutDataTypeStr=Inherit: Inherit via back propagation  PCopyOutMin=[]  PCopyOutMax=[]  NCopyOutDataTypeStr=Inherit: Inherit via back propagation  NCopyOutMin=[]  NCopyOutMax=[]  IntegratorContinuousStateAttributes=''  IntegratorStateMustResolveToSignalObject=off  IntegratorRTWStateStorageClass=Auto  FilterContinuousStateAttributes=''  FilterStateMustResolveToSignalObject=off  FilterRTWStateStorageClass=Auto  ParallelPVariant=ExternalParameters  IdealPVariant=Disabled  IVariant=ExternalParameters  DVariant=ExternalParameters  IntegratorVariant=Discrete  SatVariant=Disabled  AWVariant=Passthrough  PCopyVariant=Disabled  TRVariant=Disabled  FdbkBlocksVariant=Forward  IdealPFdbkVariant=Disabled  SatFdbkVariant=Disabled  DerivativeFilterVariant=ForwardEulerFilter  NVariant=ExternalParameters  NCopyVariant=Disabled  FilterICVariant=InternalICsFilter  IntegratorICVariant=InternalICs  ExternalResetVariant=ExternalReset  TRSumVariant=Passthrough  SumFdbkVariant=Disabled  SumVariant=Sum_PID  TsampFilterVariant=InternalTs  TsampNgainVariant=Passthrough  TsampIntegralVariant=Disabled_SignalSpec  ExternalSaturationOutDataTypeStr=Inherit: Same as second input  DerivativeSourceVariant=ErrorSignal
  Saturation1 : Saturate  UpperLimit=0  LowerLimit=-10
  SpdDiffFR : Sum  Inputs=+-  OutDataTypeStr=single  AccumDataTypeStr=single
  Switch : Switch  Criteria=u2 > Threshold  OutDataTypeStr=single  SaturateOnIntegerOverflow=off  InputSameDT=off
  LSD_TrqFR : Outport  VectorParamsAs1DForOutWhenUnconnected=off
  wires:
  Add1/1 -> Switch/1  "LSDTrqFR"
  LSD_CtrlFR/1 -> Bus Selector/1
  Switch/1 -> LSD_TrqFR/1  "LSD_TrqFR"
  Bus Selector/3 -> Switch/2  "<LSD_EnableFR>"
  EDS_TrqFR/1 -> Add1/2, Switch/3
  PID Controller/1 -> Saturation1/1  "TrqModFR"
  Bus Selector/2 -> SpdDiffFR/2  "<MotSpdActlByrpmFR>"
  Demux/3 -> PID Controller/4  "D"
  Demux/2 -> PID Controller/3  "I"
  PID_Setting/1 -> Demux/1
  Demux/5 -> PID Controller/6  "PID_Reset"
  Gain/1 -> PID Controller/1  "SpdDiffFRScaled"
  Demux/4 -> PID Controller/5  "N"
  Bus Selector/1 -> SpdDiffFR/1  "<MotSpdRefByrpmFR>"
  Demux/1 -> PID Controller/2  "P"
  SpdDiffFR/1 -> Gain/1  "SpdDiffFR"
  Saturation1/1 -> Add1/1

== system VMC_Integration/Traction_Control/LimitedSlipDifferential/PID_CtrlRL ==
  LSD_CtrlRL : Inport
  EDS_TrqRL : Inport  Port=2
  PID_Setting : Inport  Port=3
  Add1 : Sum  AccumDataTypeStr=single
  Bus Selector : BusSelector  OutputSignals=MotSpdRefByrpmRL,MotSpdActlByrpmRL,LSD_EnableRL
  Demux : Demux  Outputs=5
  Gain : Gain  Gain=0.001  ParamDataTypeStr=single  OutDataTypeStr=single
  PID Controller : slpidlib/PID Controller  Controller=PID  Form=Parallel  TimeDomain=Discrete-time  UseExternalTs=off  SampleTime=-1  IntegratorMethod=Forward Euler  FilterMethod=Forward Euler  ControllerParametersSource=external  P=500  I=0  UseKiTs=off  D=0  UseExternalDerivativeSource=off  N=100  UseFilter=on  TunerSelectOption=Transfer Function Based (PID Tuner App)  InitialConditionSource=internal  InitialConditionForIntegrator=0  InitialConditionForFilter=0  DifferentiatorICPrevScaledInput=0  ExternalReset=rising  TrackingMode=off  Kt=1  LimitOutput=off  SatLimitsSource=internal  UpperSaturationLimit=inf  LowerSaturationLimit=-inf  LinearizeAsGain=on  AntiWindupMode=none  Kb=1  LimitIntegrator=off  UpperIntegratorSaturationLimit=inf  LowerIntegratorSaturationLimit=-inf  PGainOutDataTypeStr=single  PProdOutDataTypeStr=single  POutMin=[]  POutMax=[]  IGainOutDataTypeStr=single  IProdOutDataTypeStr=single  IOutMin=[]  IOutMax=[]  DGainOutDataTypeStr=single  DProdOutDataTypeStr=single  DOutMin=[]  DOutMax=[]  NGainOutDataTypeStr=single  NProdOutDataTypeStr=single  NOutMin=[]  NOutMax=[]  SumOutDataTypeStr=single  SumOutMin=[]  SumOutMax=[]  SaturationOutMin=[]  SaturationOutMax=[]  PParamMin=[]  PParamMax=[]  IParamMin=[]  IParamMax=[]  DParamMin=[]  DParamMax=[]  NParamMin=[]  NParamMax=[]  KbParamMin=[]  KbParamMax=[]  KtParamMin=[]  KtParamMax=[]  KbOutMin=[]  KbOutMax=[]  KtOutMin=[]  KtOutMax=[]  IntegratorOutMin=[]  IntegratorOutMax=[]  FilterOutMin=[]  FilterOutMax=[]  SumI1OutMin=[]  SumI1OutMax=[]  SumI2OutMin=[]  SumI2OutMax=[]  SumI3OutMin=[]  SumI3OutMax=[]  SumI4OutMin=[]  SumI4OutMax=[]  SumDOutMin=[]  SumDOutMax=[]  DifferentiatorOutMin=[]  DifferentiatorOutMax=[]  FilterDiffOutCoefMin=[]  FilterDiffOutCoefMax=[]  ReciprocalOutMin=[]  ReciprocalOutMax=[]  SumDenOutMin=[]  SumDenOutMax=[]  SumNumOutMin=[]  SumNumOutMax=[]  DivideOutMin=[]  DivideOutMax=[]  UdiffTsProdOutMin=[]  UdiffTsProdOutMax=[]  NTsProdOutMin=[]  NTsProdOutMax=[]  UintegralTsProdOutMin=[]  UintegralTsProdOutMax=[]  UngainTsProdOutMin=[]  UngainTsProdOutMax=[]  ClampingZeroOutDataTypeStr=Inherit: Inherit via back propagation  ClampingZeroOutMin=[]  ClampingZeroOutMax=[]  FilterDenConstantOutDataTypeStr=Inherit: Inherit via back propagation  FilterDenConstantOutMin=[]  FilterDenConstantOutMax=[]  PCopyOutDataTypeStr=Inherit: Inherit via back propagation  PCopyOutMin=[]  PCopyOutMax=[]  NCopyOutDataTypeStr=Inherit: Inherit via back propagation  NCopyOutMin=[]  NCopyOutMax=[]  IntegratorContinuousStateAttributes=''  IntegratorStateMustResolveToSignalObject=off  IntegratorRTWStateStorageClass=Auto  FilterContinuousStateAttributes=''  FilterStateMustResolveToSignalObject=off  FilterRTWStateStorageClass=Auto  ParallelPVariant=ExternalParameters  IdealPVariant=Disabled  IVariant=ExternalParameters  DVariant=ExternalParameters  IntegratorVariant=Discrete  SatVariant=Disabled  AWVariant=Passthrough  PCopyVariant=Disabled  TRVariant=Disabled  FdbkBlocksVariant=Forward  IdealPFdbkVariant=Disabled  SatFdbkVariant=Disabled  DerivativeFilterVariant=ForwardEulerFilter  NVariant=ExternalParameters  NCopyVariant=Disabled  FilterICVariant=InternalICsFilter  IntegratorICVariant=InternalICs  ExternalResetVariant=ExternalReset  TRSumVariant=Passthrough  SumFdbkVariant=Disabled  SumVariant=Sum_PID  TsampFilterVariant=InternalTs  TsampNgainVariant=Passthrough  TsampIntegralVariant=Disabled_SignalSpec  ExternalSaturationOutDataTypeStr=Inherit: Same as second input  DerivativeSourceVariant=ErrorSignal
  Saturation1 : Saturate  UpperLimit=0  LowerLimit=-10
  SpdDiffRL : Sum  Inputs=+-  OutDataTypeStr=single  AccumDataTypeStr=single
  Switch : Switch  Criteria=u2 > Threshold  OutDataTypeStr=single  SaturateOnIntegerOverflow=off  InputSameDT=off
  LSD_TrqRL : Outport  VectorParamsAs1DForOutWhenUnconnected=off
  wires:
  Add1/1 -> Switch/1  "LSDTrqRL"
  LSD_CtrlRL/1 -> Bus Selector/1
  Switch/1 -> LSD_TrqRL/1  "LSD_TrqRL"
  Bus Selector/3 -> Switch/2  "<LSD_EnableRL>"
  EDS_TrqRL/1 -> Add1/2, Switch/3
  PID Controller/1 -> Saturation1/1  "TrqModRL"
  Bus Selector/2 -> SpdDiffRL/2  "<MotSpdActlByrpmRL>"
  Demux/3 -> PID Controller/4  "D"
  Demux/2 -> PID Controller/3  "I"
  PID_Setting/1 -> Demux/1
  Demux/5 -> PID Controller/6  "PID_Reset"
  Gain/1 -> PID Controller/1  "SpdDiffRLScaled"
  Demux/4 -> PID Controller/5  "N"
  Bus Selector/1 -> SpdDiffRL/1  "<MotSpdRefByrpmRL>"
  Demux/1 -> PID Controller/2  "P"
  SpdDiffRL/1 -> Gain/1  "SpdDiffRL"
  Saturation1/1 -> Add1/1

== system VMC_Integration/Traction_Control/LimitedSlipDifferential/PID_CtrlRR ==
  LSD_CtrlRR : Inport
  EDS_TrqRR : Inport  Port=2
  PID_Setting : Inport  Port=3
  Add1 : Sum  AccumDataTypeStr=single
  Bus Selector : BusSelector  OutputSignals=MotSpdRefByrpmRR,MotSpdActlByrpmRR,LSD_EnableRR
  Demux : Demux  Outputs=5
  Gain : Gain  Gain=0.001  ParamDataTypeStr=single  OutDataTypeStr=single
  PID Controller : slpidlib/PID Controller  Controller=PID  Form=Parallel  TimeDomain=Discrete-time  UseExternalTs=off  SampleTime=-1  IntegratorMethod=Forward Euler  FilterMethod=Forward Euler  ControllerParametersSource=external  P=500  I=0  UseKiTs=off  D=0  UseExternalDerivativeSource=off  N=100  UseFilter=on  TunerSelectOption=Transfer Function Based (PID Tuner App)  InitialConditionSource=internal  InitialConditionForIntegrator=0  InitialConditionForFilter=0  DifferentiatorICPrevScaledInput=0  ExternalReset=rising  TrackingMode=off  Kt=1  LimitOutput=off  SatLimitsSource=internal  UpperSaturationLimit=inf  LowerSaturationLimit=-inf  LinearizeAsGain=on  AntiWindupMode=none  Kb=1  LimitIntegrator=off  UpperIntegratorSaturationLimit=inf  LowerIntegratorSaturationLimit=-inf  PGainOutDataTypeStr=single  PProdOutDataTypeStr=single  POutMin=[]  POutMax=[]  IGainOutDataTypeStr=single  IProdOutDataTypeStr=single  IOutMin=[]  IOutMax=[]  DGainOutDataTypeStr=single  DProdOutDataTypeStr=single  DOutMin=[]  DOutMax=[]  NGainOutDataTypeStr=single  NProdOutDataTypeStr=single  NOutMin=[]  NOutMax=[]  SumOutDataTypeStr=single  SumOutMin=[]  SumOutMax=[]  SaturationOutMin=[]  SaturationOutMax=[]  PParamMin=[]  PParamMax=[]  IParamMin=[]  IParamMax=[]  DParamMin=[]  DParamMax=[]  NParamMin=[]  NParamMax=[]  KbParamMin=[]  KbParamMax=[]  KtParamMin=[]  KtParamMax=[]  KbOutMin=[]  KbOutMax=[]  KtOutMin=[]  KtOutMax=[]  IntegratorOutMin=[]  IntegratorOutMax=[]  FilterOutMin=[]  FilterOutMax=[]  SumI1OutMin=[]  SumI1OutMax=[]  SumI2OutMin=[]  SumI2OutMax=[]  SumI3OutMin=[]  SumI3OutMax=[]  SumI4OutMin=[]  SumI4OutMax=[]  SumDOutMin=[]  SumDOutMax=[]  DifferentiatorOutMin=[]  DifferentiatorOutMax=[]  FilterDiffOutCoefMin=[]  FilterDiffOutCoefMax=[]  ReciprocalOutMin=[]  ReciprocalOutMax=[]  SumDenOutMin=[]  SumDenOutMax=[]  SumNumOutMin=[]  SumNumOutMax=[]  DivideOutMin=[]  DivideOutMax=[]  UdiffTsProdOutMin=[]  UdiffTsProdOutMax=[]  NTsProdOutMin=[]  NTsProdOutMax=[]  UintegralTsProdOutMin=[]  UintegralTsProdOutMax=[]  UngainTsProdOutMin=[]  UngainTsProdOutMax=[]  ClampingZeroOutDataTypeStr=Inherit: Inherit via back propagation  ClampingZeroOutMin=[]  ClampingZeroOutMax=[]  FilterDenConstantOutDataTypeStr=Inherit: Inherit via back propagation  FilterDenConstantOutMin=[]  FilterDenConstantOutMax=[]  PCopyOutDataTypeStr=Inherit: Inherit via back propagation  PCopyOutMin=[]  PCopyOutMax=[]  NCopyOutDataTypeStr=Inherit: Inherit via back propagation  NCopyOutMin=[]  NCopyOutMax=[]  IntegratorContinuousStateAttributes=''  IntegratorStateMustResolveToSignalObject=off  IntegratorRTWStateStorageClass=Auto  FilterContinuousStateAttributes=''  FilterStateMustResolveToSignalObject=off  FilterRTWStateStorageClass=Auto  ParallelPVariant=ExternalParameters  IdealPVariant=Disabled  IVariant=ExternalParameters  DVariant=ExternalParameters  IntegratorVariant=Discrete  SatVariant=Disabled  AWVariant=Passthrough  PCopyVariant=Disabled  TRVariant=Disabled  FdbkBlocksVariant=Forward  IdealPFdbkVariant=Disabled  SatFdbkVariant=Disabled  DerivativeFilterVariant=ForwardEulerFilter  NVariant=ExternalParameters  NCopyVariant=Disabled  FilterICVariant=InternalICsFilter  IntegratorICVariant=InternalICs  ExternalResetVariant=ExternalReset  TRSumVariant=Passthrough  SumFdbkVariant=Disabled  SumVariant=Sum_PID  TsampFilterVariant=InternalTs  TsampNgainVariant=Passthrough  TsampIntegralVariant=Disabled_SignalSpec  ExternalSaturationOutDataTypeStr=Inherit: Same as second input  DerivativeSourceVariant=ErrorSignal
  Saturation1 : Saturate  UpperLimit=0  LowerLimit=-10
  SpdDiffRR : Sum  Inputs=+-  OutDataTypeStr=single  AccumDataTypeStr=single
  Switch : Switch  Criteria=u2 > Threshold  OutDataTypeStr=single  SaturateOnIntegerOverflow=off  InputSameDT=off
  LSD_TrqRR : Outport  VectorParamsAs1DForOutWhenUnconnected=off
  wires:
  Add1/1 -> Switch/1  "LSDTrqRR"
  LSD_CtrlRR/1 -> Bus Selector/1
  Switch/1 -> LSD_TrqRR/1  "LSD_TrqRR"
  Bus Selector/3 -> Switch/2  "<LSD_EnableRR>"
  EDS_TrqRR/1 -> Add1/2, Switch/3
  PID Controller/1 -> Saturation1/1  "TrqModRR"
  Bus Selector/2 -> SpdDiffRR/2  "<MotSpdActlByrpmRR>"
  Demux/3 -> PID Controller/4  "D"
  Demux/2 -> PID Controller/3  "I"
  PID_Setting/1 -> Demux/1
  Demux/5 -> PID Controller/6  "PID_Reset"
  Gain/1 -> PID Controller/1  "SpdDiffRRScaled"
  Demux/4 -> PID Controller/5  "N"
  Bus Selector/1 -> SpdDiffRR/1  "<MotSpdRefByrpmRR>"
  Demux/1 -> PID Controller/2  "P"
  SpdDiffRR/1 -> Gain/1  "SpdDiffRR"
  Saturation1/1 -> Add1/1
